simulink model "my_pv_sys_fpga_rtlab"  (Simulink 8.4)
settings: Solver=ode3  SolverMode=SingleTasking  StartTime=0.0  StopTime=inf  FixedStep=Ts  RelTol=1e-3
PostLoadFcn:
  | Ts = 20e-6;
InitFcn:
  | Ts = 20e-6;
undefined symbols (not defined in the file): SW01
libraries: powerlib_meascontrol x8, simulink x4, rteventslib x4, rtlab x3, rtio_opalrt_common x2, cpuconverter_lib x1
settings Model: ARTEMISmethode_block_infos=$$__separator__$$  Creator=PYRobert  LastModifiedBy=jiang  BufferReuse=off
settings DataIOCC: SaveOutput=off  SignalLogging=off  SaveTime=off  SignalLoggingName=sigsOut
settings OptimizationCC: BlockReduction=off  OptimizeBlockIOStorage=off  BufferReuse=off  GlobalBufferReuse=off  ExpressionFolding=off  LocalBlockOutputs=off  InitFltsAndDblsToZero=on
settings DebuggingCC: SaveWithParameterizedLinksMsg=none  SignalResolutionControl=TryResolveAllWithWarning  SolverPrmCheckMsg=none  MultiTaskDSMMsg=warning  MultiTaskCondExecSysMsg=none  StrictBusMsg=None
settings HardwareCC: TargetEndianess=LittleEndian  TargetHWDeviceType=MATLAB Host  ProdEqTarget=off
settings RTWCC: IncludeERTFirstTime=on
settings GRTTargetCC: TargetFcnLib=ansi_tfl_tmw.mat
settings ConfigurationSet: Description=SimMechanics 2G

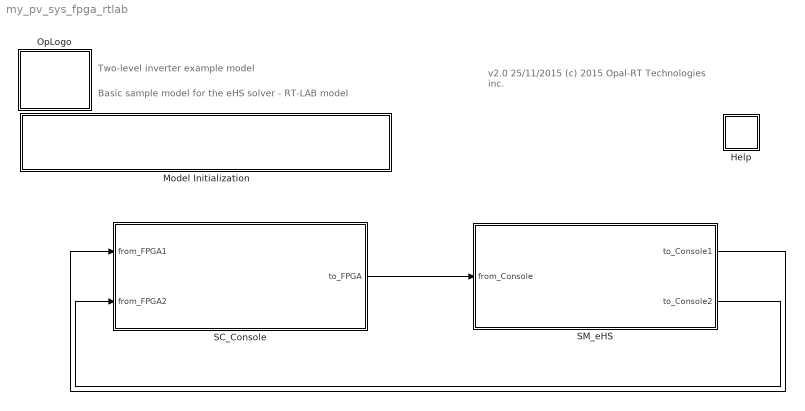
== system my_pv_sys_fpga_rtlab ==
  note: v2.0 25/11/2015
      | (c) 2015 Opal-RT Technologies inc.
  note: Two-level inverter example model
  note: Basic sample model for the eHS solver - RT-LAB model
  Help : Subsystem  mask(OpDoc){docfile=../Help/help.html}
      mask init:
      | %patch([1,1,0,0,.8,1],[.8,0,0,1,1,.8],[.8 .8 .8]);
      | %patch([.15 .78 .78 .15 .15],[.8 .8 .83 .83 .8],[.9 .9 .9]);
      | %patch([.15 .78 .78 .15 .15],[.7 .7 .73 .73 .8],[.9 .9 .9]);
      | %patch([.15 .78 .78 .15 .15],[.6 .6 .63 .63 .6],[.9 .9 .9]);
      | %patch([.15 .78 .78 .15 .15],[.5 .5 .53 .53 .5],[.9 .9 .9]);
      | %patch([.15 .78 .78 .15 .15],[.4 .4 .43 .43 .4],[.9 .9 .9]);
      settings: OpenFcn=OpHelp_cb(gcb);
      mask Display: image(imread('opdoc.bmp'))
  Model Initialization : Subsystem  mask(Model Functions){InitFcnX=Ts = 20e-6;, prel=off, posl=on, inif=on, strf=off}
      mask prompts: InitFcnX "Initialisation"; prel "Preload Function"; posl "PostLoad Function"; inif "InitFcn"; strf "StartFcn"
      mask init:
      | currentBlock = gcb;
      | root = bdroot(currentBlock);
      | 
      | if ~strcmp(get_param(root,'BlockDiagramType'),'library')
      |     if prel==1
      |         set_param(root, 'PreLoadFcn', InitFcnX);
      |     else
      |         set_param(root, 'PreLoadFcn', '');
      |     end
      |     if inif==1
      |         set_param(root, 'InitFcn', InitFcnX);
      |     else
      |         set_param(root, 'InitFcn', '');
      |     end
      |     if strf==1
      |         set_param(root, 'StartFcn', InitFcnX);
      |     else
      |         set_param(root, 'StartFcn', '');
      |     end
      |     if posl==1
      |         set_param(root, 'PostLoadFcn', InitFcnX);
      |     else
      |         set_param(root, 'PostLoadFcn', '');
      |     end
      | end
      | 
      | pos = get_param(currentBlock, 'Position');
      | width = pos(3) - pos(1); height = pos(4) - pos(2);
      | txt = [ upper(root) '\n' '- InitFcn. . . . . '  get_param(root, 'InitFcn') ];
      settings: CopyFcn=set_param(gcb,'LinkStatus','none')
      mask Display: text(5, height*0.5, txt, 'horizontalAlignment', 'left', 'verticalAlignment', 'middle') ;
  OpLogo : Subsystem
      mask Display:
      | opLogo = imread('efsOpLogo.tif','tif');
      | image(opLogo(:,:,1:3));
  SC_Console : Subsystem
  SM_eHS : Subsystem
  wires:
  SC_Console/1(to_FPGA) -> SM_eHS/1(from_Console)
  SM_eHS/1(to_Console1) -> SC_Console/1(from_FPGA1)
  SM_eHS/2(to_Console2) -> SC_Console/2(from_FPGA2)

== system my_pv_sys_fpga_rtlab/Help ==

== system my_pv_sys_fpga_rtlab/Model Initialization ==

== system my_pv_sys_fpga_rtlab/OpLogo ==

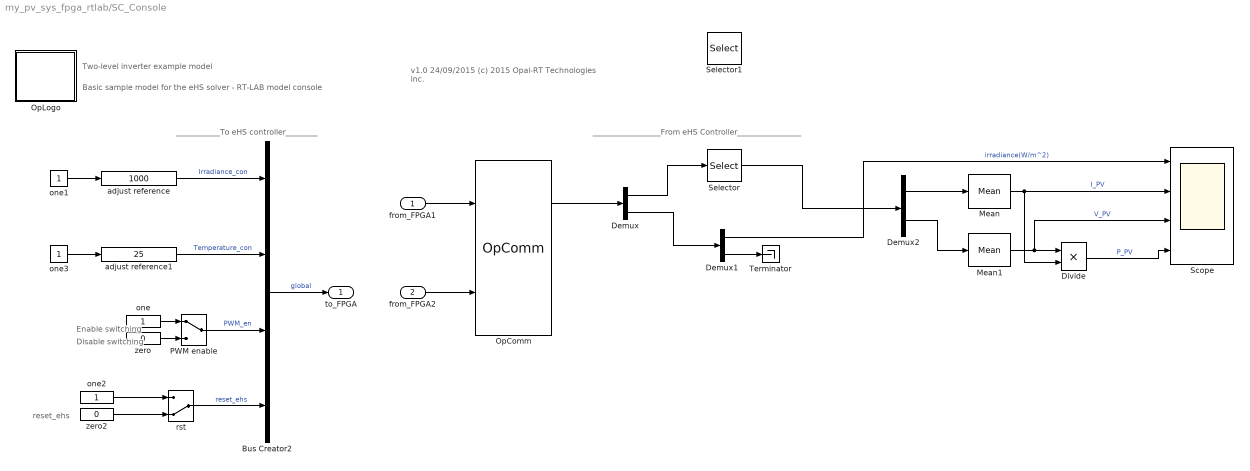
== system my_pv_sys_fpga_rtlab/SC_Console ==
  note: ___________To eHS controller________
  note: _________________From eHS Controller________________
  note: Enable switching
  note: Disable switching
  note: v1.0 24/09/2015
      | (c) 2015 Opal-RT Technologies inc.
  note: Two-level inverter example model
  note: Basic sample model for the eHS solver - RT-LAB model console
  note: reset_ehs
  from_FPGA1 : Inport
  from_FPGA2 : Inport  Port=2
  Bus Creator2 : BusCreator
  Demux : Demux  Outputs=2
  Demux1 : Demux  Outputs=2
  Demux2 : Demux  Outputs=2
  Divide : Product  Inputs=**
  Mean : powerlib_meascontrol/Measurements/Mean  Freq=50  Vinit=0  Ts=0
  Mean1 : powerlib_meascontrol/Measurements/Mean  Freq=50  Vinit=0  Ts=0
  OpComm : rtlab/OpComm  nbport=2  groupe_acq=1  subsys_rate=0  st=0  Synchronization=off  Interpolation=on  Threshold=1.0  Missed_Data=off  Sim_Time=off  Samples=off  dynSigOut=off  from_console=0  warning_done=off  writeOpCommFile=off  Offset=off
  OpLogo : Subsystem
      mask Display:
      | opLogo = imread('efsOpLogo.tif','tif');
      | image(opLogo(:,:,1:3));
  PWM enable : ManualSwitch
  Scope : Scope  NumInputPorts=4
      settings: YMin=-5~-5~-5~-5  YMax=5~5~5~5
  Selector : Selector  Indices=[1 2]
  Selector1 : Selector  Indices=[1 2]
  Terminator : Terminator
  adjust reference : simulink/Math Operations/Slider Gain  low=0  gain=1000  high=1000
  adjust reference1 : simulink/Math Operations/Slider Gain  low=0  gain=25  high=60
  one{,1..3} (4 alike) : Constant
  rst : ManualSwitch  CurrentSetting=0
  zero : Constant  Value=0
  zero2 : Constant  Value=0
  to_FPGA : Outport
  wires:
  Bus Creator2/1 -> to_FPGA/1  "global"
  PWM enable/1 -> Bus Creator2/3  "PWM_en"
  zero/1 -> PWM enable/2
  one/1 -> PWM enable/1
  rst/1 -> Bus Creator2/4  "reset_ehs"
  zero2/1 -> rst/2
  one2/1 -> rst/1
  from_FPGA1/1 -> OpComm/1
  from_FPGA2/1 -> OpComm/2
  one1/1 -> adjust reference/1
  one3/1 -> adjust reference1/1
  adjust reference/1 -> Bus Creator2/1  "Irradiance_con"
  adjust reference1/1 -> Bus Creator2/2  "Temperature_con"
  OpComm/1 -> Demux/1
  Demux/1 -> Selector/1
  Demux/2 -> Demux1/1
  Demux1/2 -> Terminator/1
  Selector/1 -> Demux2/1
  Demux1/1 -> Scope/1  "irradiance(W/m^2)"
  Demux2/1 -> Mean/1
  Demux2/2 -> Mean1/1
  Mean/1 -> Divide/2, Scope/2  "I_PV"
  Mean1/1 -> Divide/1, Scope/3  "V_PV"
  Divide/1 -> Scope/4  "P_PV"

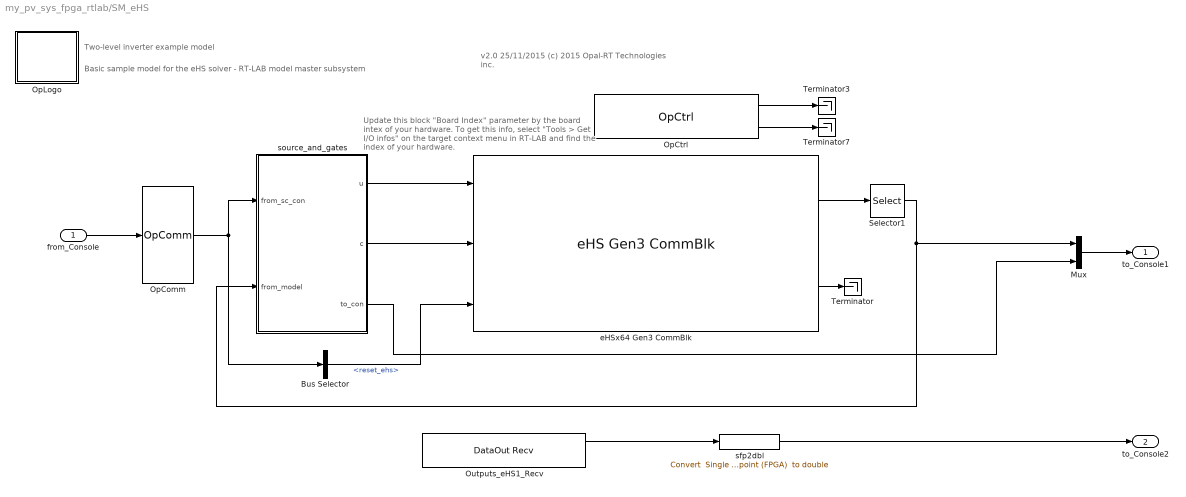
== system my_pv_sys_fpga_rtlab/SM_eHS ==
  note: v2.0 25/11/2015
      | (c) 2015 Opal-RT Technologies inc.
  note: Two-level inverter example model
  note: Basic sample model for the eHS solver - RT-LAB model master subsystem
  note: Update this block "Board Index" parameter by the
      | board intex of your hardware. To get this info, select
      | "Tools > Get I/O infos" on the target context menu
      | in RT-LAB and find the index of your hardware.
  from_Console : Inport
  Bus Selector : BusSelector  OutputSignals=reset_ehs
  Mux : Mux  Inputs=2
  OpComm : rtlab/OpComm  nbport=1  groupe_acq=1  subsys_rate=0  st=0  Synchronization=on  Interpolation=on  Threshold=1.0  Missed_Data=off  Sim_Time=off  Samples=off  dynSigOut=off  from_console=1  warning_done=off  writeOpCommFile=off  Offset=off
  OpCtrl : rtio_opalrt_common/OpCtrl  CtrlName='eHS Ctrl'  boardid=0  BitstreamFilename=MMPK7_1-EX-0001-2_3_2_19-300Series_eHSgen3_with_IOs-303-03.bin  numconfig=-1  mode=Master  externalClock=off  decimRtsi=0  calibIO=off  SampleTime=0  loadinport=-1  BoardType=MMPK7  SecondaryPresent=off  sync_type=Audio
  OpLogo : Subsystem
      mask Display:
      | opLogo = imread('efsOpLogo.tif','tif');
      | image(opLogo(:,:,1:3));
  Outputs_eHS1_Recv : rtio_opalrt_common/DataOut Recv  CtrlName='eHS Ctrl'  FcnNos=2  width=7  portType=uint32  sampleTime=0  checkVersion=off  expectedId=0  expectedVersion=0  opComp=>=
      settings: AttributesFormatString=%<CtrlName>
  Selector1 : Selector  Indices=[1:7]
  Terminator : Terminator
  Terminator3 : Terminator
  Terminator7 : Terminator
  eHSx64 Gen3 CommBlk : cpuconverter_lib/eHS Gen3 CommBlk  GenMat=off  solver_size=x64  circuit_mtx1=my_pv_sys_fpga  Ts_eHS_1_explicit=on  Ts_eHS_1=2.5e-07  SimeHS1=off  ShowAdv1=on  gs1=0.5  v_init1=zeros(1,4)  i_init1=zeros(1,4)  netlist_name=my_pv_sys_fpga.mdl  ts_min=2.05e-07  nb_u=3  input_names=|  nb_sw=4  switches_names=SW01-04_01 | SW01-04_02 | SW01-04_03 | SW01-04_04  nb_y=7  output_names=Y01 IPANEL I | Y02 VPANEL U | Y03 VPH U | Y04 VINV U | Y05 IGRID I | Y06 VGRID U | Y07 IG I  nb_nsd=12  Input_config1_popup=Constant from RT-LAB block (all)  input_config_1="[zeros(32,1)  (0:31)']"  input_nb_auto=on  input_nb=3  UseSWG=off  SWGPortNbs=3  Pulse_ctrl1_popup=From RT-LAB block (all)  GateCtrlSelPanel=off  Pulse_ctrl1=[zeros(72,1) (0:71)']  Polarity1_popup=Active-high (all)  Polarity1=zeros(1,72)  pulse_nb=8  rte_pulse_nb=SW01-08  nb_event=4  static_pulse=none  scn_en=off  xls_file=diode_bridge.xls  scn_cmd=do nothing  xls_page=1  nscn_max=102  nscn_used=1  scn_log_en=on  CtrlName='eHS Ctrl'  Ts=Ts  PortNbs=[1 2 1 2:1:2+8 1]  blkid1=0
      | U01
      | 14,400 V | U02 IPH
      |  | U03 ID
      settings: AttributesFormatString=%<CtrlName>
  sfp2dbl : rtlab/Miscellaneous/Convert  Single floating-point (FPGA)  to double
  source_and_gates : Subsystem
  to_Console1 : Outport
  to_Console2 : Outport  Port=2
  wires:
  from_Console/1 -> OpComm/1
  OpComm/1 -> Bus Selector/1, source_and_gates/1(from_sc_con)
  OpCtrl/1 -> Terminator3/1
  OpCtrl/2 -> Terminator7/1
  source_and_gates/1(u) -> eHSx64 Gen3 CommBlk/1
  source_and_gates/2(c) -> eHSx64 Gen3 CommBlk/2
  Selector1/1 -> Mux/1, source_and_gates/2(from_model)
  sfp2dbl/1 -> to_Console2/1
  eHSx64 Gen3 CommBlk/2 -> Terminator/1
  eHSx64 Gen3 CommBlk/1 -> Selector1/1
  Outputs_eHS1_Recv/1 -> sfp2dbl/1
  Bus Selector/1 -> eHSx64 Gen3 CommBlk/3  "<reset_ehs>"
  source_and_gates/3(to_con) -> Mux/2
  Mux/1 -> to_Console1/1

== system my_pv_sys_fpga_rtlab/SC_Console/OpLogo ==

== system my_pv_sys_fpga_rtlab/SM_eHS/OpLogo ==

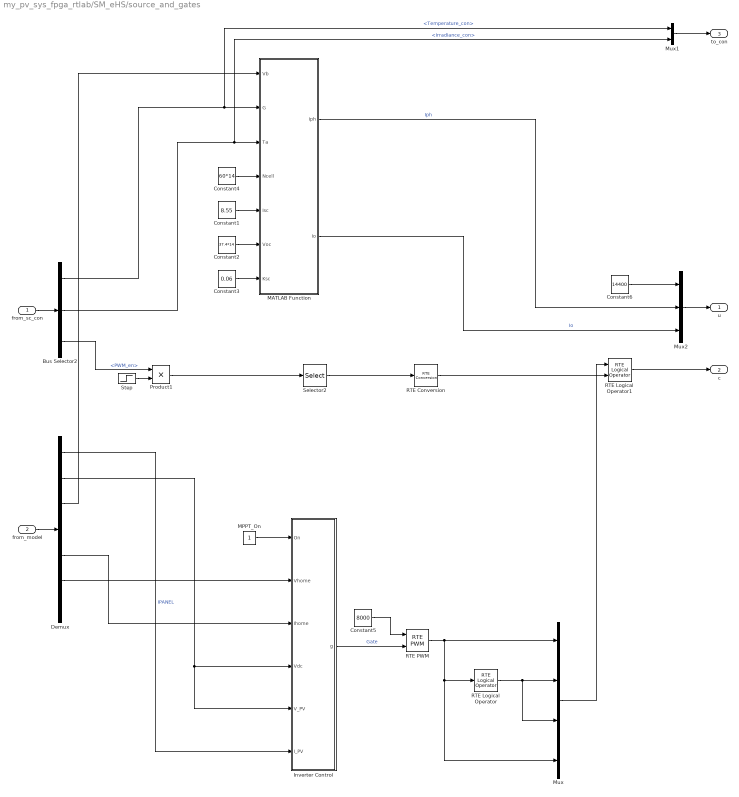
== system my_pv_sys_fpga_rtlab/SM_eHS/source_and_gates ==
  from_sc_con : Inport
  from_model : Inport  Port=2
  Bus Selector2 : BusSelector  OutputSignals=Temperature_con,Irradiance_con,PWM_en
  Constant1 : Constant  Value=8.55
  Constant2 : Constant  Value=37.4*14
  Constant3 : Constant  Value=0.06
  Constant4 : Constant  Value=60*14
  Constant5 : Constant  Value=8000
  Constant6 : Constant  Value=14400
  Demux : Demux  Outputs=7
  Inverter Control : Subsystem  mask(Inverter Control){Pnom=3500, Fnom=50, Vnom_prim=240, Vnom_dc=400, Increment_MPPT=0.003, Limits_MPPT=[ 450 375 ], Vdc_ref_Init=425, Kp_VDCreg=12, Ki_VDCreg=200, Kp_Ireg=0.15, Ki_Ireg=6.6, RLff=[ 0.002 0.20 ], Fc=8000, PWMmode12=Bipolar, Ts_Control=50e-6, Ts_PWMgenerator=50e-6}
      mask prompts: Pnom "Power (VA)"; Fnom "Frequency (Hz)"; Vnom_prim "Primary voltage (Vrms LL)"; Vnom_dc "DC voltage (V)"; Increment_MPPT "Output increment (V)"; Limits_MPPT "Output limits [ Upper  Lower ]"; Vdc_ref_Init "Output initial value (V)"; Kp_VDCreg "Proportional gain"; Ki_VDCreg "Integral gain"; Kp_Ireg "Proportional gain"; Ki_Ireg "Integral gain"; RLff "Feedforward Values [Rff Lff] (pu)"; Fc "Carrier frequency (Hz)"; PWMmode12 "PWM method"; Ts_Control "Control systems"; Ts_PWMgenerator "PWM generator"
      mask help:
      | The main components of the Inverter Control are:
      | 1. PLL & Measurements
      | 2. Maximum Power Point Tracker System (MPPT) using a Perturb & Observe algorithm
      | 3. DC Voltage Regulator
      | 4. Current Regulator
      | 5. PWM Modulator
      mask TypeOptions PWMmode12: Unipolar | Bipolar
  MATLAB Function : MATLAB Function  TreatAsAtomicUnit=on
  MPPT_On : Constant
  Mux : Mux
  Mux1 : Mux  Inputs=2
  Mux2 : Mux  Inputs=3
  Product1 : Product  RndMeth=Zero
  RTE Conversion : rteventslib/Signal Attributes/RTE Conversion  inputdatatype=Double  outputdatatype=RTE Boolean  compensation=Enabled  nbMaxEvents=4  sampleTime=Ts
  RTE Logical Operator : rteventslib/Math Operations/RTE Logical Operator  LogicalOperator=NOT  NbrInput=1  NbrMaxEvents=10
  RTE Logical Operator1 : rteventslib/Math Operations/RTE Logical Operator  LogicalOperator=AND  NbrInput=2  NbrMaxEvents=4
  RTE PWM : rteventslib/Sources/RTE PWM  ShiftedTransition=Enabled  MaxEvents=10  SampleTime=Ts
  Selector2 : Selector  InputPortWidth=1  Indices=[ones(1,4)*1]
  Step : Step  Time=0.1  SampleTime=Ts
  u : Outport
  c : Outport  Port=2
  to_con : Outport  Port=3
  wires:
  Bus Selector2/3 -> Product1/1  "<PWM_en>"
  Step/1 -> Product1/2
  Selector2/1 -> RTE Conversion/1
  RTE Conversion/1 -> RTE Logical Operator1/2
  Product1/1 -> Selector2/1
  Mux2/1 -> u/1
  from_sc_con/1 -> Bus Selector2/1
  Bus Selector2/1 -> Mux1/1, MATLAB Function/2(G)  "<Temperature_con>"
  Bus Selector2/2 -> Mux1/2, MATLAB Function/3(Ta)  "<Irradiance_con>"
  MPPT_On/1 -> Inverter Control/1(On)
  Constant4/1 -> MATLAB Function/4(Ncell)
  Constant1/1 -> MATLAB Function/5(Isc)
  Constant2/1 -> MATLAB Function/6(Voc)
  Constant3/1 -> MATLAB Function/7(Ksc)
  from_model/1 -> Demux/1
  Demux/1 -> Inverter Control/6(I_PV)  "IPANEL"
  Demux/3 -> MATLAB Function/1(Vb)
  Demux/2 -> Inverter Control/4(Vdc), Inverter Control/5(V_PV)
  Demux/6 -> Inverter Control/2(Vhome)
  Demux/5 -> Inverter Control/3(Ihome)
  Constant5/1 -> RTE PWM/1
  Inverter Control/1(g) -> RTE PWM/2  "Gate"
  RTE PWM/1 -> RTE Logical Operator/1, Mux/4, Mux/1
  RTE Logical Operator/1 -> Mux/2, Mux/3
  Mux/1 -> RTE Logical Operator1/1
  RTE Logical Operator1/1 -> c/1
  Constant6/1 -> Mux2/1
  MATLAB Function/2(Io) -> Mux2/3  "Io"
  MATLAB Function/1(Iph) -> Mux2/2  "Iph"
  Mux1/1 -> to_con/1

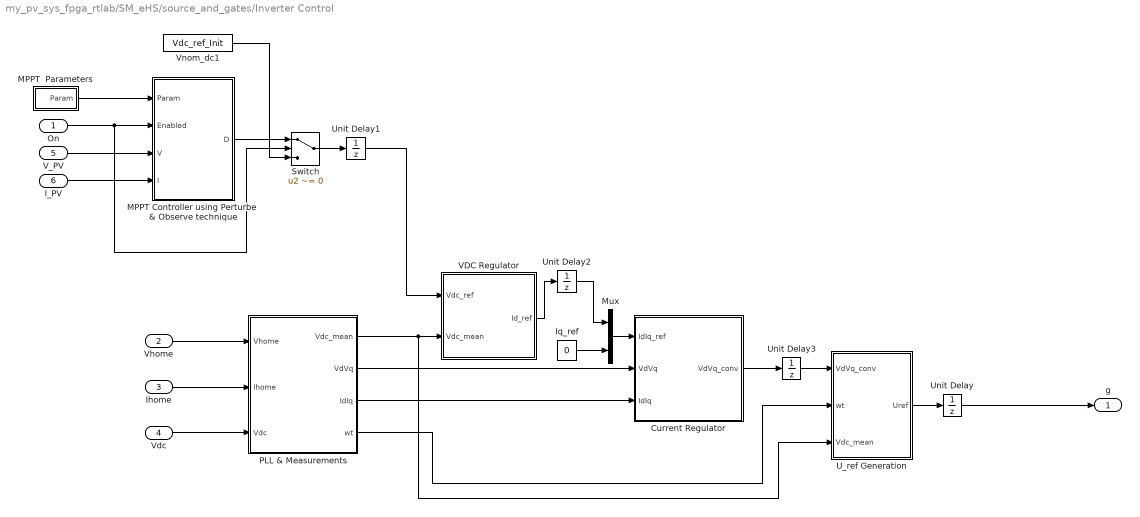
== system my_pv_sys_fpga_rtlab/SM_eHS/source_and_gates/Inverter Control ==
  On : Inport  PortDimensions=1
  Vhome : Inport  Port=2  PortDimensions=1
  Ihome : Inport  Port=3  PortDimensions=1
  Vdc : Inport  Port=4  PortDimensions=1
  V_PV : Inport  Port=5  PortDimensions=1
  I_PV : Inport  Port=6  PortDimensions=1
  Current Regulator : Subsystem
  Iq_ref : Constant  Value=0
  MPPT  Parameters : Subsystem
  "MPPT Controller using Perturbe  & Observe technique  " : MATLAB Function  TreatAsAtomicUnit=on
  Mux : Mux  Inputs=2
  PLL & Measurements : Subsystem
  Switch : Switch  Criteria=u2 ~= 0
  "U_ref Generation " : Subsystem
  Unit Delay : UnitDelay  InitialCondition=0.1684  SampleTime=Ts_Control
  Unit Delay1 : UnitDelay  SampleTime=Ts_Control
  Unit Delay2 : UnitDelay  SampleTime=Ts_Control
  Unit Delay3 : UnitDelay  SampleTime=Ts_Control
  VDC Regulator : Subsystem
  Vnom_dc1 : Constant  Value=Vdc_ref_Init
  g : Outport
  wires:
  Iq_ref/1 -> Mux/2
  Vhome/1 -> PLL & Measurements/1(Vhome)
  Ihome/1 -> PLL & Measurements/2(Ihome)
  V_PV/1 -> "MPPT Controller using Perturbe  & Observe technique  "/3(V)
  I_PV/1 -> "MPPT Controller using Perturbe  & Observe technique  "/4(I)
  MPPT  Parameters/1(Param) -> "MPPT Controller using Perturbe  & Observe technique  "/1(Param)
  On/1 -> "MPPT Controller using Perturbe  & Observe technique  "/2(Enabled), Switch/2
  "MPPT Controller using Perturbe  & Observe technique  "/1(D) -> Switch/1
  Vdc/1 -> PLL & Measurements/3(Vdc)
  Vnom_dc1/1 -> Switch/3
  PLL & Measurements/2(VdVq) -> Current Regulator/2(VdVq)
  PLL & Measurements/3(IdIq) -> Current Regulator/3(IdIq)
  Mux/1 -> Current Regulator/1(IdIq_ref)
  PLL & Measurements/1(Vdc_mean) -> "U_ref Generation "/3(Vdc_mean), VDC Regulator/2(Vdc_mean)
  PLL & Measurements/4(wt) -> "U_ref Generation "/2(wt)
  "U_ref Generation "/1(Uref) -> Unit Delay/1
  Switch/1 -> Unit Delay1/1
  Unit Delay1/1 -> VDC Regulator/1(Vdc_ref)
  VDC Regulator/1(Id_ref) -> Unit Delay2/1
  Unit Delay2/1 -> Mux/1
  Current Regulator/1(VdVq_conv) -> Unit Delay3/1
  Unit Delay3/1 -> "U_ref Generation "/1(VdVq_conv)
  Unit Delay/1 -> g/1

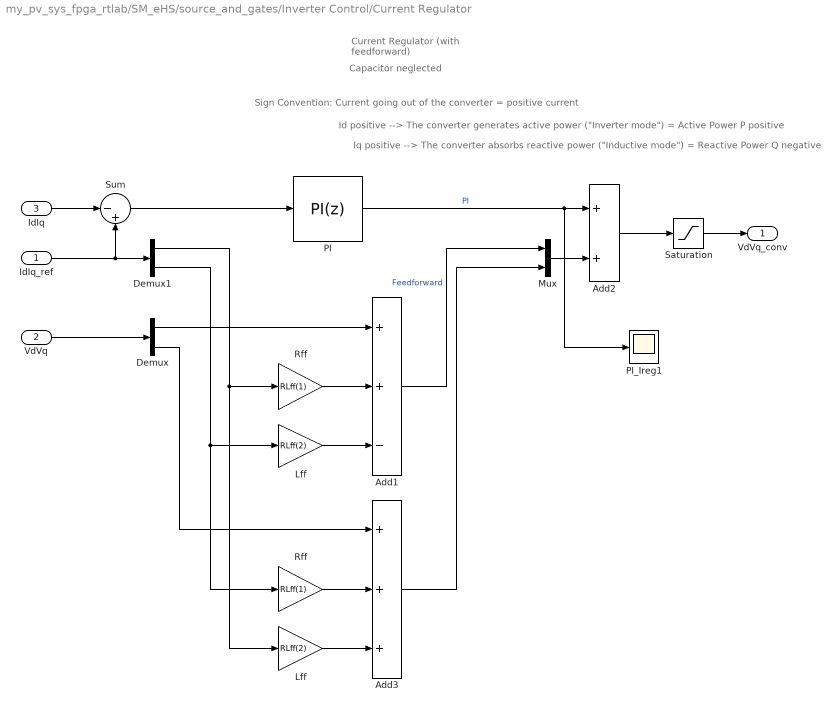
== system my_pv_sys_fpga_rtlab/SM_eHS/source_and_gates/Inverter Control/Current Regulator ==
  note: Id positive --> The converter generates active power ("Inverter mode") = Active Power P positive
  note: Iq positive --> The converter absorbs reactive power ("Inductive mode") = Reactive Power Q negative
  note: Sign Convention: Current going out of the converter = positive current
  note: Current Regulator
      | (with feedforward)
  note: Capacitor neglected
  IdIq_ref : Inport  PortDimensions=2
  VdVq : Inport  Port=2  PortDimensions=2
  IdIq : Inport  Port=3  PortDimensions=2
  Add1 : Sum  Inputs=++-
  Add2 : Sum
  Add3 : Sum  Inputs=+++
  Demux : Demux  Outputs=2
  Demux1 : Demux  Outputs=2
  Lff : Gain  Gain=RLff(2)  SaturateOnIntegerOverflow=on  OutDataTypeStr=Inherit: Same as input  ParamDataTypeStr=Inherit: Same as input
  "Lff  " : Gain  Gain=RLff(2)  SaturateOnIntegerOverflow=on  OutDataTypeStr=Inherit: Same as input  ParamDataTypeStr=Inherit: Same as input
  Mux : Mux  Inputs=2
  PI : simulink/Continuous/PID Controller  Controller=PI  TimeDomain=Discrete-time  SampleTime=Ts_Control  IntegratorMethod=Forward Euler  FilterMethod=Forward Euler  Form=Parallel  P=Kp_Ireg  I=Ki_Ireg  D=0  N=100  InitialConditionSource=internal  InitialConditionForIntegrator=0  InitialConditionForFilter=0  ExternalReset=none  LimitOutput=on  UpperSaturationLimit=1.5  LowerSaturationLimit=-1.5  LinearizeAsGain=off  AntiWindupMode=none  Kb=1  TrackingMode=off  Kt=1  PParamMin=[]  PParamMax=[]  IParamMin=[]  IParamMax=[]  DParamMin=[]  DParamMax=[]  NParamMin=[]  NParamMax=[]  KbParamMin=[]  KbParamMax=[]  KtParamMin=[]  KtParamMax=[]  POutMin=[]  POutMax=[]  IOutMin=[]  IOutMax=[]  DOutMin=[]  DOutMax=[]  NOutMin=[]  NOutMax=[]  KbOutMin=[]  KbOutMax=[]  KtOutMin=[]  KtOutMax=[]  IntegratorOutMin=[]  IntegratorOutMax=[]  FilterOutMin=[]  FilterOutMax=[]  SumOutMin=[]  SumOutMax=[]  SumI1OutMin=[]  SumI1OutMax=[]  SumI2OutMin=[]  SumI2OutMax=[]  SumI3OutMin=[]  SumI3OutMax=[]  SumDOutMin=[]  SumDOutMax=[]  SaturationOutMin=[]  SaturationOutMax=[]  IntegratorContinuousStateAttributes=''  IntegratorStateMustResolveToSignalObject=off  IntegratorRTWStateStorageClass=Auto  FilterContinuousStateAttributes=''  FilterStateMustResolveToSignalObject=off  FilterRTWStateStorageClass=Auto  DifferentiatorICPrevScaledInput=0  DifferentiatorOutMin=[]  DifferentiatorOutMax=[]  UseFilter=on
  PI_Ireg1 : Scope
      settings: YMin=-0.25  YMax=0.45
  Rff : Gain  Gain=RLff(1)  SaturateOnIntegerOverflow=on  OutDataTypeStr=Inherit: Same as input  ParamDataTypeStr=Inherit: Same as input
  "Rff " : Gain  Gain=RLff(1)  SaturateOnIntegerOverflow=on  OutDataTypeStr=Inherit: Same as input  ParamDataTypeStr=Inherit: Same as input
  Saturation : Saturate  UpperLimit=1.5  LowerLimit=-1.5
  Sum : Sum  Inputs=|-+
  VdVq_conv : Outport
  wires:
  Add3/1 -> Mux/2
  Demux/2 -> Add3/1
  Add1/1 -> Mux/1  "Feedforward"
  Lff/1 -> Add3/3
  Rff/1 -> Add3/2
  Demux1/2 -> Rff/1, "Lff  "/1
  "Lff  "/1 -> Add1/3
  Demux1/1 -> Lff/1, "Rff "/1
  "Rff "/1 -> Add1/2
  Demux/1 -> Add1/1
  VdVq/1 -> Demux/1
  Saturation/1 -> VdVq_conv/1
  Add2/1 -> Saturation/1
  IdIq/1 -> Sum/1
  IdIq_ref/1 -> Demux1/1, Sum/2
  Sum/1 -> PI/1
  PI/1 -> Add2/1, PI_Ireg1/1  "PI"
  Mux/1 -> Add2/2

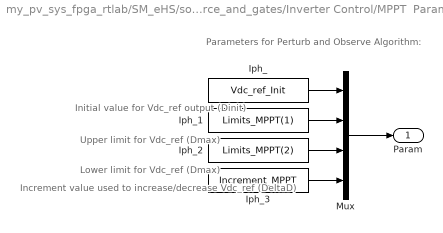
== system my_pv_sys_fpga_rtlab/SM_eHS/source_and_gates/Inverter Control/MPPT  Parameters ==
  note: Upper limit for Vdc_ref (Dmax)
  note: Increment value used to increase/decrease Vdc_ref (DeltaD)
  note: Initial value for Vdc_ref output (Dinit)
  note: Lower limit for Vdc_ref (Dmax)
  note: Parameters for Perturb and Observe Algorithm:
  Iph_ : Constant  Value=Vdc_ref_Init
  Iph_1 : Constant  Value=Limits_MPPT(1)
  Iph_2 : Constant  Value=Limits_MPPT(2)
  Iph_3 : Constant  Value=Increment_MPPT
  Mux : Mux
  Param : Outport
  wires:
  Iph_/1 -> Mux/1
  Iph_1/1 -> Mux/2
  Iph_2/1 -> Mux/3
  Iph_3/1 -> Mux/4
  Mux/1 -> Param/1

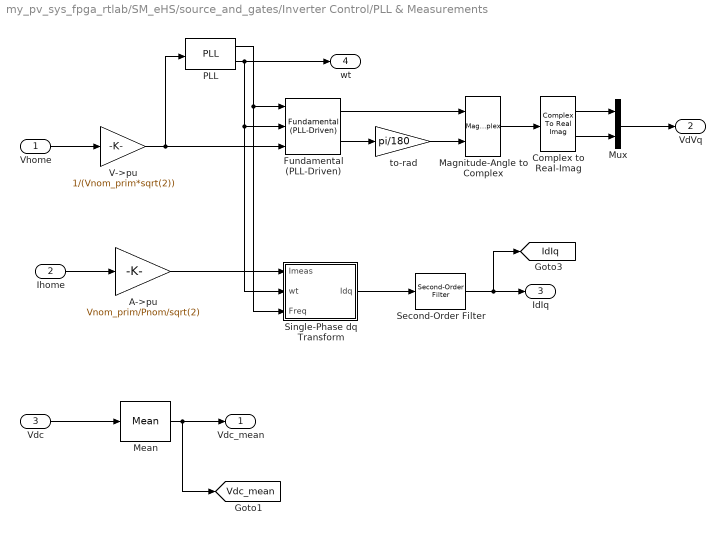
== system my_pv_sys_fpga_rtlab/SM_eHS/source_and_gates/Inverter Control/PLL & Measurements ==
  Vhome : Inport
  Ihome : Inport  Port=2
  Vdc : Inport  Port=3
  A->pu : Gain  Gain=Vnom_prim/Pnom/sqrt(2)  SaturateOnIntegerOverflow=on  OutDataTypeStr=Inherit: Same as input  ParamDataTypeStr=Inherit: Same as input
  Complex to Real-Imag : ComplexToRealImag
  Fundamental (PLL-Driven) : powerlib_meascontrol/Measurements/Fundamental (PLL-Driven)  Finit=Fnom  Fmin=45  InInit=[1, 0]  Ts=Ts_Control
  Magnitude-Angle to Complex : MagnitudeAngleToComplex
  Mean : powerlib_meascontrol/Measurements/Mean  Freq=Fnom  Vinit=Vdc_ref_Init  Ts=Ts_Control
  Mux : Mux  Inputs=2
  PLL : powerlib_meascontrol/PLL/PLL  Fmin=40  Par_Init=[0, Fnom]  ParK=[180, 3200, 1]  TcD=1e-4  MaxRateChangeFreq=12  FilterCutOffFreq=25  Ts=Ts_Control  AGC=on
  Second-Order Filter : powerlib_meascontrol/Filters/Second-Order Filter  FilterType=Lowpass  Fo=2000  Zeta=1  Ts=Ts_Control  Initialize=on  Vac_Init="[0,  0,  60;0,0,60]"  Vdc_Init=[0.9 0]  PlotResponse=off  FreqRange=[0, 500, 1]
  Single-Phase dq Transform : Subsystem
  V->pu : Gain  Gain=1/(Vnom_prim*sqrt(2))  SaturateOnIntegerOverflow=on  OutDataTypeStr=Inherit: Same as input  ParamDataTypeStr=Inherit: Same as input
  to-rad : Gain  Gain=pi/180
  Vdc_mean : Outport
  VdVq : Outport  Port=2
  IdIq : Outport  Port=3
  wt : Outport  Port=4
  tag scope: IdIq=global, Vdc_mean=global
  wires:
  Mean/1 -> Vdc_mean/1, [Vdc_mean]
  Vdc/1 -> Mean/1
  to-rad/1 -> Magnitude-Angle to Complex/2
  Mux/1 -> VdVq/1
  Complex to Real-Imag/2 -> Mux/2
  Complex to Real-Imag/1 -> Mux/1
  Magnitude-Angle to Complex/1 -> Complex to Real-Imag/1
  Fundamental (PLL-Driven)/2 -> to-rad/1
  Fundamental (PLL-Driven)/1 -> Magnitude-Angle to Complex/1
  A->pu/1 -> Single-Phase dq Transform/1(Imeas)
  PLL/1 -> Single-Phase dq Transform/3(Freq), Fundamental (PLL-Driven)/1
  PLL/2 -> wt/1, Fundamental (PLL-Driven)/2, Single-Phase dq Transform/2(wt)
  Ihome/1 -> A->pu/1
  Vhome/1 -> V->pu/1
  V->pu/1 -> Fundamental (PLL-Driven)/3, PLL/1
  Single-Phase dq Transform/1(Idq) -> Second-Order Filter/1
  Second-Order Filter/1 -> [IdIq], IdIq/1

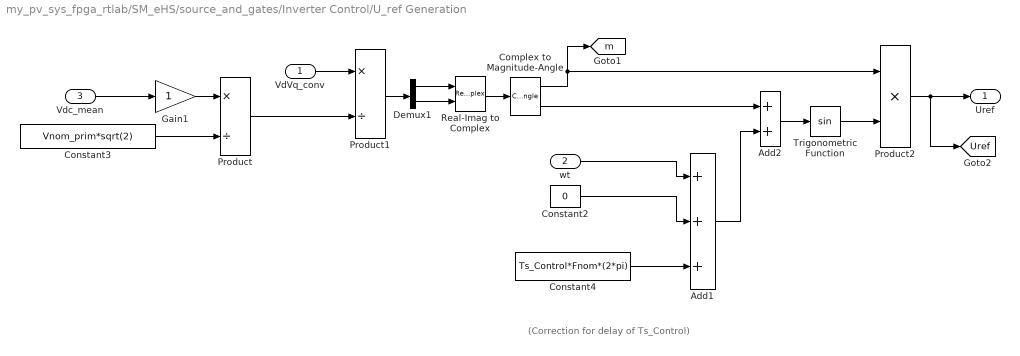
== system my_pv_sys_fpga_rtlab/SM_eHS/source_and_gates/Inverter Control/U_ref Generation  ==
  note: (Correction for delay of Ts_Control)
  VdVq_conv : Inport
  wt : Inport  Port=2
  Vdc_mean : Inport  Port=3
  Add1 : Sum  Inputs=+++
  Add2 : Sum
  Complex to Magnitude-Angle : ComplexToMagnitudeAngle
  Constant2 : Constant  Value=0
  Constant3 : Constant  Value=Vnom_prim*sqrt(2)
  Constant4 : Constant  Value=Ts_Control*Fnom*(2*pi)
  Demux1 : Demux  Outputs=2
  Gain1 : Gain
  Product : Product  Inputs=*/  RndMeth=Zero
  Product1 : Product  Inputs=*/  RndMeth=Zero
  Product2 : Product  Inputs=**  RndMeth=Zero
  Real-Imag to Complex : RealImagToComplex
  Trigonometric Function : Trigonometry
  Uref : Outport
  tag scope: Uref=global, m=global
  wires:
  VdVq_conv/1 -> Product1/1
  Product2/1 -> Uref/1, [Uref]
  Vdc_mean/1 -> Gain1/1
  Constant4/1 -> Add1/3
  wt/1 -> Add1/1
  Trigonometric Function/1 -> Product2/2
  Complex to Magnitude-Angle/1 -> [m], Product2/1
  Add2/1 -> Trigonometric Function/1
  Add1/1 -> Add2/2
  Complex to Magnitude-Angle/2 -> Add2/1
  Product/1 -> Product1/2
  Constant3/1 -> Product/2
  Constant2/1 -> Add1/2
  Demux1/2 -> Real-Imag to Complex/2
  Demux1/1 -> Real-Imag to Complex/1
  Real-Imag to Complex/1 -> Complex to Magnitude-Angle/1
  Gain1/1 -> Product/1
  Product1/1 -> Demux1/1

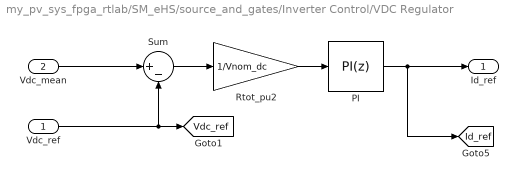
== system my_pv_sys_fpga_rtlab/SM_eHS/source_and_gates/Inverter Control/VDC Regulator ==
  Vdc_ref : Inport  PortDimensions=1
  Vdc_mean : Inport  Port=2  PortDimensions=1
  PI : simulink/Continuous/PID Controller  Controller=PI  TimeDomain=Discrete-time  SampleTime=Ts_Control  IntegratorMethod=Trapezoidal  FilterMethod=Forward Euler  Form=Parallel  P=Kp_VDCreg  I=Ki_VDCreg  D=0  N=100  InitialConditionSource=internal  InitialConditionForIntegrator=0.9226  InitialConditionForFilter=0  ExternalReset=none  LimitOutput=on  UpperSaturationLimit=1.5  LowerSaturationLimit=-1.5  LinearizeAsGain=off  AntiWindupMode=none  Kb=1  TrackingMode=off  Kt=1  PParamMin=[]  PParamMax=[]  IParamMin=[]  IParamMax=[]  DParamMin=[]  DParamMax=[]  NParamMin=[]  NParamMax=[]  KbParamMin=[]  KbParamMax=[]  KtParamMin=[]  KtParamMax=[]  POutMin=[]  POutMax=[]  IOutMin=[]  IOutMax=[]  DOutMin=[]  DOutMax=[]  NOutMin=[]  NOutMax=[]  KbOutMin=[]  KbOutMax=[]  KtOutMin=[]  KtOutMax=[]  IntegratorOutMin=[]  IntegratorOutMax=[]  FilterOutMin=[]  FilterOutMax=[]  SumOutMin=[]  SumOutMax=[]  SumI1OutMin=[]  SumI1OutMax=[]  SumI2OutMin=[]  SumI2OutMax=[]  SumI3OutMin=[]  SumI3OutMax=[]  SumDOutMin=[]  SumDOutMax=[]  SaturationOutMin=[]  SaturationOutMax=[]  IntegratorContinuousStateAttributes=''  IntegratorStateMustResolveToSignalObject=off  IntegratorRTWStateStorageClass=Auto  FilterContinuousStateAttributes=''  FilterStateMustResolveToSignalObject=off  FilterRTWStateStorageClass=Auto  DifferentiatorICPrevScaledInput=0  DifferentiatorOutMin=[]  DifferentiatorOutMax=[]  UseFilter=on
  Rtot_pu2 : Gain  Gain=1/Vnom_dc  SaturateOnIntegerOverflow=on  OutDataTypeStr=Inherit: Same as input  ParamDataTypeStr=Inherit: Same as input
  Sum : Sum  Inputs=|+-
  Id_ref : Outport  InitialOutput=0
  tag scope: Id_ref=global, Vdc_ref=global
  wires:
  Rtot_pu2/1 -> PI/1
  Vdc_ref/1 -> Sum/2, [Vdc_ref]
  Vdc_mean/1 -> Sum/1
  Sum/1 -> Rtot_pu2/1
  PI/1 -> Id_ref/1, [Id_ref]

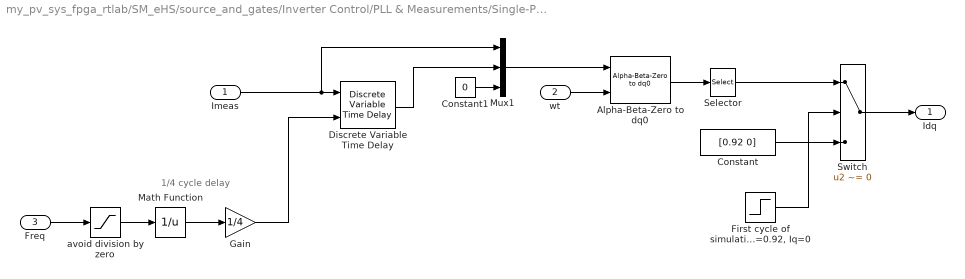
== system my_pv_sys_fpga_rtlab/SM_eHS/source_and_gates/Inverter Control/PLL & Measurements/Single-Phase dq Transform ==
  note: 1/4 cycle delay
  Imeas : Inport
  wt : Inport  Port=2
  Freq : Inport  Port=3
  Alpha-Beta-Zero to dq0 : powerlib_meascontrol/Transformations/Alpha-Beta-Zero to dq0  Alignment=90 degrees behind phase A axis
  Constant : Constant  Value=[0.92 0]
  Constant1 : Constant  Value=0
  Discrete Variable Time Delay : powerlib_meascontrol/Additional Components/Discrete Variable Time Delay  MaxDelay=1  InitialValue=0  Ts=Ts_Control  DFT=on
  "First cycle of simulation Id=0.92, Iq=0" : Step  Time=1/Fnom  SampleTime=Ts_Control
  Gain : Gain  Gain=1/4
  Math Function : Math  Operator=reciprocal  SaturateOnIntegerOverflow=on
  Mux1 : Mux  Inputs=3
  Selector : Selector  InputPortWidth=3  Indices=[1 2]
  Switch : Switch  Criteria=u2 ~= 0
  avoid division by zero : Saturate  UpperLimit=70  LowerLimit=40
  Idq : Outport
  wires:
  Constant1/1 -> Mux1/3
  Discrete Variable Time Delay/1 -> Mux1/2
  Mux1/1 -> Alpha-Beta-Zero to dq0/1
  Imeas/1 -> Discrete Variable Time Delay/1, Mux1/1
  wt/1 -> Alpha-Beta-Zero to dq0/2
  Alpha-Beta-Zero to dq0/1 -> Selector/1
  Freq/1 -> avoid division by zero/1
  avoid division by zero/1 -> Math Function/1
  Math Function/1 -> Gain/1
  Gain/1 -> Discrete Variable Time Delay/2
  Selector/1 -> Switch/1
  Switch/1 -> Idq/1
  Constant/1 -> Switch/3
  "First cycle of simulation Id=0.92, Iq=0"/1 -> Switch/2

== matlab function SM_eHS/source_and_gates/MATLAB Function ==
  data: Vb input double; Iph output double; G input double; Ta input double; Ncell input double; Isc input double; Voc input double; Ksc input double; Io output double
function [Iph, Io] = PVpanel_new(Vb, G, Ta, Ncell, Isc, Voc, Ksc)

    toKelvin = 273;
    Ksc = Ksc / 100;
    G_ref = 1000;
    Ta_ref = 25 + toKelvin;
    Ta = Ta + toKelvin;
    deltaT = Ta - Ta_ref;
    k = 1.381e-23;
    q = 1.6e-19;
    eg = 1.12;                  % bandgap energy(1.12 eV)
    A = 1.3;                    % ideal factor
    a = Ncell * k * A * Ta / q;
    a_ref = Ncell * k * A * Ta_ref / q;
    Iph_ref = Isc;
    Voc_ref = Voc;
    Iph = G / G_ref * Iph_ref * (1 + Ksc * deltaT);
    Io_ref = Iph_ref / (exp(Voc_ref / a_ref) - 1);
    Io = Io_ref * (Ta / Ta_ref)^3 * ...
        exp((q * eg / A / k) * (1/Ta_ref - 1/Ta));
    Io = Io * (exp(Vb / a) - 1);

end

== matlab function SM_eHS/source_and_gates/Inverter Control/MPPT Controller using Perturbe & Observe technique  ==
  settings: updateMethod=DISCRETE  sampleTime=Ts_Control
  data: Param input double; Enabled input double; V input double; I input double; D output double
function D  = PandO(Param, Enabled, V, I)

% MPPT controller based on the Perturb & Observe algorithm.

% D output = Reference for DC link voltage (Vdc_ref) 
%
% Enabled input = 1 to enable the MPPT controller
% V input = PV array terminal voltage (V)
% I input = PV array current (A)
%
% Param input:
Dinit = Param(1);  %Initial value for Vdc_ref
Dmax = Param(2);   %Maximum value for Vdc_ref
Dmin = Param(3);   %Minimum value for Vdc_ref
deltaD = Param(4); %Increment value used to increase/decrease Vdc_ref
%  

persistent Vold Pold Dold;

dataType = 'double';

if isempty(Vold)
    Vold=0;
    Pold=0;
    Dold=Dinit;
end
P= V*I;
dV= V - Vold;
dP= P - Pold;

if dP ~= 0 & Enabled ~=0
    if dP < 0
        if dV < 0
            D = Dold + deltaD;
        else
            D = Dold - deltaD;
        end
    else
        if dV < 0
            D = Dold - deltaD;
        else
            D = Dold + deltaD;
        end    
    end
else D=Dold;
end

if D >= Dmax | D<= Dmin
    D=Dold;
end

Dold=D;
Vold=V;
Pold=P;
